simulink model "ANN_Sim"  (R2024a)
settings: Solver=ode4  StartTime=0.0  StopTime=5  FixedStep=50e-6  RelTol=1e-3
PreLoadFcn:
  | Rs=0.02;
  | Ls=0.4;
  | Sm=0.2205;
  | p=4;
  | J=0.006;
  | B=0;
  | f=60;
  | 
  | intialSpeed = 0;
  | speedChange = 200;
  | loadTorque = 0;
  | Vdc = 500;
  | samplingTime = 50;
libraries: slpidlib x1
settings Model: Creator=Windows10  LastModifiedBy=anugr
settings SolverCC: AlgebraicLoopSolver=TrustRegion
settings DataIOCC: ReturnWorkspaceOutputs=off
settings DebuggingCC: UnconnectedInputMsg=warning  UnconnectedOutputMsg=warning  UnconnectedLineMsg=warning  UnderSpecifiedDimensionMsg=warning
settings ModelReferenceCC: EnableRefExpFcnMdlSchedulingChecks=on
settings RTWCC: GPUComputeCapability=3.5

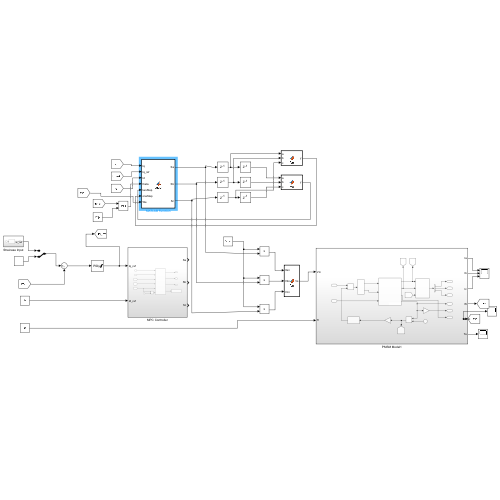
[thumbnail: Simulink's stored preview of the top-level diagram]
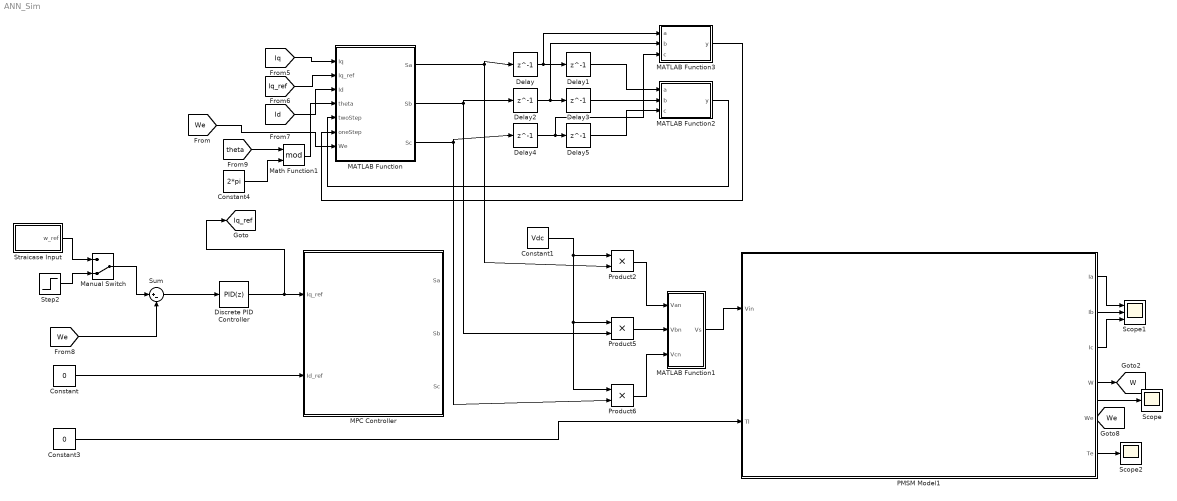
== system ANN_Sim ==
  Constant : Constant  Value=0
  Constant1 : Constant  Value=Vdc
  Constant3 : Constant  Value=0
  Constant4 : Constant  Value=2*pi
  Delay{,1..5} (6 alike) : Delay  DelayLength=1
  Discrete PID Controller : slpidlib/PID Controller  Controller=PID  Form=Parallel  TimeDomain=Discrete-time  UseExternalTs=off  SampleTime=-1  IntegratorMethod=Forward Euler  FilterMethod=Forward Euler  ControllerParametersSource=internal  P=1  I=0.1  UseKiTs=off  D=0.1  UseExternalDerivativeSource=off  N=100  UseFilter=off  TunerSelectOption=Transfer Function Based (PID Tuner App)  InitialConditionSource=internal  InitialConditionForIntegrator=0  InitialConditionForFilter=0  DifferentiatorICPrevScaledInput=0  ExternalReset=none  TrackingMode=off  Kt=1  LimitOutput=on  SatLimitsSource=internal  UpperSaturationLimit=90  LowerSaturationLimit=-90  LinearizeAsGain=on  AntiWindupMode=clamping  Kb=1  LimitIntegrator=off  UpperIntegratorSaturationLimit=inf  LowerIntegratorSaturationLimit=-inf  POutMin=[]  POutMax=[]  IOutMin=[]  IOutMax=[]  DOutMin=[]  DOutMax=[]  NOutMin=[]  NOutMax=[]  SumOutMin=[]  SumOutMax=[]  SaturationOutMin=[]  SaturationOutMax=[]  PParamMin=[]  PParamMax=[]  IParamMin=[]  IParamMax=[]  DParamMin=[]  DParamMax=[]  NParamMin=[]  NParamMax=[]  KbParamMin=[]  KbParamMax=[]  KtParamMin=[]  KtParamMax=[]  KbOutMin=[]  KbOutMax=[]  KtOutMin=[]  KtOutMax=[]  IntegratorOutMin=[]  IntegratorOutMax=[]  FilterOutMin=[]  FilterOutMax=[]  SumI1OutMin=[]  SumI1OutMax=[]  SumI2OutMin=[]  SumI2OutMax=[]  SumI3OutMin=[]  SumI3OutMax=[]  SumI4OutMin=[]  SumI4OutMax=[]  SumDOutMin=[]  SumDOutMax=[]  DifferentiatorOutMin=[]  DifferentiatorOutMax=[]  FilterDiffOutCoefMin=[]  FilterDiffOutCoefMax=[]  ReciprocalOutMin=[]  ReciprocalOutMax=[]  SumDenOutMin=[]  SumDenOutMax=[]  SumNumOutMin=[]  SumNumOutMax=[]  DivideOutMin=[]  DivideOutMax=[]  UdiffTsProdOutMin=[]  UdiffTsProdOutMax=[]  NTsProdOutMin=[]  NTsProdOutMax=[]  UintegralTsProdOutMin=[]  UintegralTsProdOutMax=[]  UngainTsProdOutMin=[]  UngainTsProdOutMax=[]  ClampingZeroOutDataTypeStr=Inherit: Inherit via back propagation  ClampingZeroOutMin=[]  ClampingZeroOutMax=[]  FilterDenConstantOutDataTypeStr=Inherit: Inherit via back propagation  FilterDenConstantOutMin=[]  FilterDenConstantOutMax=[]  PCopyOutDataTypeStr=Inherit: Inherit via back propagation  PCopyOutMin=[]  PCopyOutMax=[]  NCopyOutDataTypeStr=Inherit: Inherit via back propagation  NCopyOutMin=[]  NCopyOutMax=[]  IntegratorContinuousStateAttributes=''  IntegratorStateMustResolveToSignalObject=off  IntegratorRTWStateStorageClass=Auto  FilterContinuousStateAttributes=''  FilterStateMustResolveToSignalObject=off  FilterRTWStateStorageClass=Auto  ParallelPVariant=InternalParameters  IdealPVariant=Disabled  IVariant=InternalParameters  DVariant=InternalParameters  IntegratorVariant=Discrete  SatVariant=Enabled  AWVariant=DiscClampingParallel  PCopyVariant=Disabled  TRVariant=Disabled  FdbkBlocksVariant=Forward  IdealPFdbkVariant=Disabled  SatFdbkVariant=Disabled  DerivativeFilterVariant=Differentiator  NVariant=Passthrough  NCopyVariant=Disabled_SignalSpec  FilterICVariant=InternalICsDifferentiator  IntegratorICVariant=InternalICs  ExternalResetVariant=Disabled  TRSumVariant=Passthrough  SumFdbkVariant=Disabled  SumVariant=Sum_PID  TsampFilterVariant=InternalTs  TsampNgainVariant=Passthrough  TsampIntegralVariant=Disabled_SignalSpec  ExternalSaturationOutDataTypeStr=Inherit: Same as second input  DerivativeSourceVariant=ErrorSignal
  MATLAB Function : MATLAB Function  TreatAsAtomicUnit=on
  MATLAB Function1 : MATLAB Function  TreatAsAtomicUnit=on
  MATLAB Function2 : MATLAB Function  TreatAsAtomicUnit=on
  MATLAB Function3 : MATLAB Function  TreatAsAtomicUnit=on
  MPC Controller : Subsystem
  Manual Switch : ManualSwitch  CurrentSetting=0
  Math Function1 : Math  Operator=mod
  PMSM Model1 : Subsystem
  Product2 : Product
  Product5 : Product
  Product6 : Product
  Scope : Scope
  Scope1 : Scope  NumInputPorts=3
  Scope2 : Scope
  Step2 : Step  Time=2.5  Before=200  After=400  SampleTime=0
  Straicase Input : Subsystem
  Sum : Sum  Inputs=|+-
  tag scope: Iq_ref=global, W=global, We=global
  wires:
  Step2/1 -> Manual Switch/2
  Manual Switch/1 -> Sum/1
  Straicase Input/1(w_ref) -> Manual Switch/1
  PMSM Model1/3(Ic) -> Scope1/3
  PMSM Model1/6(Te) -> Scope2/1
  PMSM Model1/5(We) -> Scope/1, [We]
  Constant/1 -> MPC Controller/2(Id_ref)
  Constant3/1 -> PMSM Model1/2(Tl)
  PMSM Model1/2(Ib) -> Scope1/2
  MATLAB Function1/1(Vs) -> PMSM Model1/1(Vin)
  Product6/1 -> MATLAB Function1/3(Vcn)
  PMSM Model1/1(Ia) -> Scope1/1
  PMSM Model1/4(W) -> [W]
  Discrete PID Controller/1 -> [Iq_ref], MPC Controller/1(Iq_ref)
  Product2/1 -> MATLAB Function1/1(Van)
  [We] -> Sum/2
  Constant1/1 -> Product5/1, Product6/1, Product2/1
  Sum/1 -> Discrete PID Controller/1
  Product5/1 -> MATLAB Function1/2(Vbn)
  [theta] -> Math Function1/1
  Math Function1/1 -> MATLAB Function/4(theta)
  Constant4/1 -> Math Function1/2
  [Iq] -> MATLAB Function/1(Iq)
  [Iq_ref] -> MATLAB Function/2(Iq_ref)
  [Id] -> MATLAB Function/3(Id)
  MATLAB Function/1(Sa) -> Delay/1, Product2/2
  Delay/1 -> MATLAB Function3/1(a), Delay1/1
  Delay2/1 -> MATLAB Function3/2(b), Delay3/1
  MATLAB Function/2(Sb) -> Delay2/1, Product5/2
  Delay4/1 -> MATLAB Function3/3(c), Delay5/1
  MATLAB Function/3(Sc) -> Delay4/1, Product6/2
  Delay3/1 -> MATLAB Function2/2(b)
  Delay1/1 -> MATLAB Function2/1(a)
  Delay5/1 -> MATLAB Function2/3(c)
  MATLAB Function3/1(y) -> MATLAB Function/6(oneStep)
  MATLAB Function2/1(y) -> MATLAB Function/5(twoStep)
  [We] -> MATLAB Function/7(We)

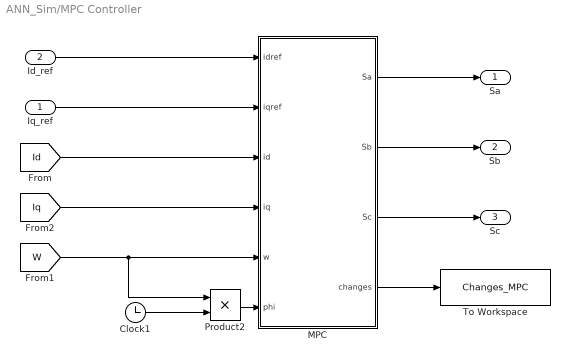
== system ANN_Sim/MPC Controller ==
  Iq_ref : Inport
  Id_ref : Inport  Port=2
  Clock1 : Clock
  MPC : MATLAB Function  TreatAsAtomicUnit=on
  Product2 : Product
  To Workspace : ToWorkspace  VariableName=Changes_MPC  SaveFormat=Timeseries  SampleTime=-1
  Sa : Outport
  Sb : Outport  Port=2
  Sc : Outport  Port=3
  wires:
  [Iq] -> MPC/4(iq)
  [W] -> MPC/5(w), Product2/1
  MPC/3(Sc) -> Sc/1
  [Id] -> MPC/3(id)
  Id_ref/1 -> MPC/1(idref)
  Iq_ref/1 -> MPC/2(iqref)
  Product2/1 -> MPC/6(phi)
  Clock1/1 -> Product2/2
  MPC/2(Sb) -> Sb/1
  MPC/1(Sa) -> Sa/1
  MPC/4(changes) -> To Workspace/1

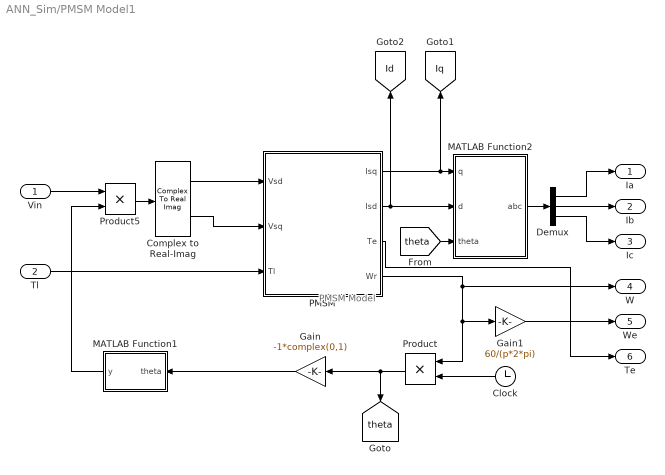
== system ANN_Sim/PMSM Model1 ==
  note: PMSM Model
  Vin : Inport
  Tl : Inport  Port=2
  Clock : Clock
  Complex to Real-Imag : ComplexToRealImag
  Demux : Demux  Outputs=3
  Gain : Gain  Gain=-1*complex(0,1)
  Gain1 : Gain  Gain=60/(p*2*pi)
  MATLAB Function1 : MATLAB Function  TreatAsAtomicUnit=on
  MATLAB Function2 : MATLAB Function  TreatAsAtomicUnit=on
  PMSM : Subsystem
  Product : Product
  Product5 : Product
  Ia : Outport
  Ib : Outport  Port=2
  Ic : Outport  Port=3
  W : Outport  Port=4
  We : Outport  Port=5
  Te : Outport  Port=6
  tag scope: Id=global, Iq=global, theta=global
  wires:
  Tl/1 -> PMSM/3(Tl)
  PMSM/4(Wr) -> W/1, Gain1/1, Product/1
  Product/1 -> Gain/1, [theta]
  Demux/3 -> Ic/1
  Clock/1 -> Product/2
  PMSM/1(Isq) -> [Iq], MATLAB Function2/1(q)
  MATLAB Function1/1(y) -> Product5/2
  Complex to Real-Imag/1 -> PMSM/1(Vsd)
  PMSM/3(Te) -> Te/1
  PMSM/2(Isd) -> MATLAB Function2/2(d), [Id]
  Complex to Real-Imag/2 -> PMSM/2(Vsq)
  Product5/1 -> Complex to Real-Imag/1
  Gain/1 -> MATLAB Function1/1(theta)
  Demux/1 -> Ia/1
  MATLAB Function2/1(abc) -> Demux/1
  Vin/1 -> Product5/1
  Gain1/1 -> We/1
  Demux/2 -> Ib/1
  [theta] -> MATLAB Function2/3(theta)

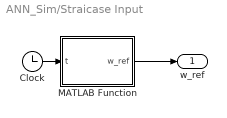
== system ANN_Sim/Straicase Input ==
  Clock : Clock
  MATLAB Function : MATLAB Function  TreatAsAtomicUnit=on
  w_ref : Outport
  wires:
  Clock/1 -> MATLAB Function/1(t)
  MATLAB Function/1(w_ref) -> w_ref/1

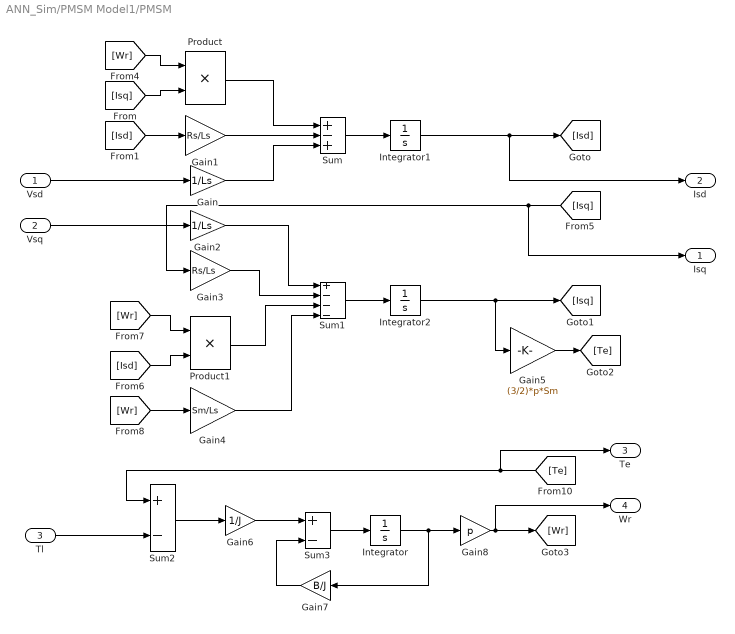
== system ANN_Sim/PMSM Model1/PMSM ==
  Vsd : Inport
  Vsq : Inport  Port=2
  Tl : Inport  Port=3
  Gain : Gain  Gain=1/Ls
  Gain1 : Gain  Gain=Rs/Ls
  Gain2 : Gain  Gain=1/Ls
  Gain3 : Gain  Gain=Rs/Ls
  Gain4 : Gain  Gain=Sm/Ls
  Gain5 : Gain  Gain=(3/2)*p*Sm
  Gain6 : Gain  Gain=1/J
  Gain7 : Gain  Gain=B/J
  Gain8 : Gain  Gain=p
  Integrator : Integrator
  Integrator1 : Integrator
  Integrator2 : Integrator
  Product : Product
  Product1 : Product
  Sum : Sum  Inputs=+-+
  Sum1 : Sum  Inputs=+---
  Sum2 : Sum  Inputs=+-
  Sum3 : Sum  Inputs=+-
  Isq : Outport
  Isd : Outport  Port=2
  Te : Outport  Port=3
  Wr : Outport  Port=4
  wires:
  Gain5/1 -> [Te]
  [Wr] -> Gain4/1
  [Isq] -> Isq/1, Gain3/1
  [Te] -> Te/1, Sum2/1
  Integrator2/1 -> Gain5/1, [Isq]
  Gain6/1 -> Sum3/1
  Sum1/1 -> Integrator2/1
  Gain/1 -> Sum/3
  Integrator/1 -> Gain8/1, Gain7/1
  Tl/1 -> Sum2/2
  Gain8/1 -> Wr/1, [Wr]
  Gain2/1 -> Sum1/1
  Sum3/1 -> Integrator/1
  Vsd/1 -> Gain/1
  Sum2/1 -> Gain6/1
  [Isd] -> Product1/2
  Gain7/1 -> Sum3/2
  Gain3/1 -> Sum1/2
  Gain4/1 -> Sum1/4
  [Wr] -> Product/1
  [Isq] -> Product/2
  Product1/1 -> Sum1/3
  [Wr] -> Product1/1
  Product/1 -> Sum/1
  Gain1/1 -> Sum/2
  [Isd] -> Gain1/1
  Sum/1 -> Integrator1/1
  Vsq/1 -> Gain2/1
  Integrator1/1 -> Isd/1, [Isd]

== matlab function ANN_Sim/MATLAB Function ==
  data: Iq input; Sa output; Iq_ref input; Id input; theta input; Sb output; Sc output; twoStep input; oneStep input; We input
function [Sa, Sb, Sc] = ANN(Iq, Iq_ref, Id, theta, twoStep, oneStep, We)
Sa = 0; Sb = 0; Sc = 0;
u = [Iq; Iq_ref; Id; sin(theta); cos(theta); twoStep; oneStep];
y = myANN(u);
[~, state] = max(y);
state = state - 1;

switch state
    case 0
        Sa = 0; Sb = 0; Sc = 0;
    case 1
        Sa = 0; Sb = 0; Sc = 1;
    case 2
        Sa = 0; Sb = 1; Sc = 0;
    case 3
        Sa = 0; Sb = 1; Sc = 1;
    case 4
        Sa = 1; Sb = 0; Sc = 0;
    case 5
        Sa = 1; Sb = 0; Sc = 1;
    case 6
        Sa = 1; Sb = 1; Sc = 0;
    case 7
        Sa = 1; Sb = 1; Sc = 1;
end

end

== matlab function ANN_Sim/Straicase Input/MATLAB Function ==
  data: t input; w_ref output
function w_ref = speed_ref(t)
%#codegen
step = 10;      % speed increment
holdT = 0.6;    % hold time
w_ref = step * (floor(t/holdT) + 1);
end

== matlab function ANN_Sim/MPC Controller/MPC ==
  settings: updateMethod=DISCRETE
  data: idref input; Sa output; iqref input; id input; iq input; w input; Sb output; Sc output; phi input; changes output
function [Sa, Sb, Sc, changes] = mpc(idref, iqref, id, iq, w,phi) 
    %% Initialisation 
    R = 0.02;
    Ls = 0.4;
    Vdc = 400;
    Lambda_f = 0.2205;
    Ts = 1e-6;
    imax=80;
    p=4;
    cost=1e14; 
    persistent state; 
    if isempty(state) 
        state = 1; 
    end
    S = [0 0 0; 1 0 0; 1 1 0; 0 1 0; 0 1 1; 0 0 1; 1 0 1; 1 1 1]; 
    prev_state = state;
    for i=1:8
    ud = Vdc*(2/3)*(S(i,1)*cos(phi) + S(i,2)*cos(phi-2*pi/3) + S(i,3)*cos(phi + 2*pi/3)); 
    uq = Vdc*(2/3)* (-S(i,1) *sin(phi) - S(i,2)*sin(phi- 2*pi/3) - S(i,3)*sin(phi + 2*pi/3));
    id1 = ((1 -(R*Ts)/Ls)*id) + ((Ts*ud)/Ls) + (w*Ts*iq) ; 
    iq1 = ((1 - (R*Ts)/Ls)*iq) + ((Ts*uq)/Ls) - ((w*Ts*id)) - (((w*Ts*Lambda_f)/Ls)); 
    f = 0; 
    if abs(id1) > imax || abs(iq1) > imax 
        f = 1e14; 
    end
    current_cost=(idref-id1)^2 + (iqref-iq1)^2 +f; 
    if(current_cost<cost) 
        state=i;
        cost=current_cost;
    end
          
    end
    changes = sum(S(state,:) ~= S(prev_state,:));
    Sa = S(state,1);
    Sb = S(state,2); 
    Sc = S(state,3);
end

== matlab function ANN_Sim/MATLAB Function2 ==
  data: a input; y output; b input; c input
function y = fcn(a, b, c)

y = 4 * a + 2 * b + c;

== matlab function ANN_Sim/MATLAB Function3 ==
  data: a input; y output; b input; c input
function y = fcn(a, b, c)

y = 4 * a + 2 * b + c;

== matlab function ANN_Sim/MATLAB Function1 ==
  data: Van input; Vs output; Vbn input; Vcn input
function Vs = fcn(Van,Vbn,Vcn)

a=complex(cos(2*pi/3),sin(2*pi/3)); 
Vs =(2/3)*(Van+(a*Vbn)+((a^2)*Vcn)) ;

== matlab function ANN_Sim/PMSM Model1/MATLAB Function1 ==
  data: theta input; y output
function y = fcn(theta)

y = exp((theta));

== matlab function ANN_Sim/PMSM Model1/MATLAB Function2 ==
  data: q input; d input; abc output; theta input
function abc = dq_to_abc(q, d, theta)
    % Inputs:
    % d, q   : DQ components
    % theta  : Electrical angle in radians

    % Transformation matrix
    T = [cos(theta), -sin(theta), 1; 
         cos(theta - 2*pi/3), -sin(theta - 2*pi/3), 1; 
         cos(theta + 2*pi/3), -sin(theta + 2*pi/3), 1];

    % Calculate abc components
    abc = (2/3) * T * [d; q; 0];
end
